simulink model "FieldOrientedControl_Model"  (R2024b)
settings: Solver=FixedStepAuto  StartTime=0.0  StopTime=10.0  FixedStep=1e-07  RelTol=1e-3
InitFcn:
  | clear all;
  | clc;
  | Start_Run;
values from neighbouring files (symbols this model uses):
  dq_decouping_ena = Simulink.Parameter    [FOC_Data.m]
  dq_voltage_ratio = Simulink.Parameter    [FOC_Data.m]
  duty_sat_lower = Simulink.Parameter    [FOC_Data.m]
  duty_sat_upper = Simulink.Parameter    [FOC_Data.m]
  I_s_max = Simulink.Parameter    [FOC_Data.m]
  KI_c = Simulink.Parameter    [FOC_Data.m]
  KI_w = Simulink.Parameter    [FOC_Data.m]
  Kp_c = Simulink.Parameter    [FOC_Data.m]
  Kp_w = Simulink.Parameter    [FOC_Data.m]
  L_d = Simulink.Parameter    [FOC_Data.m]
  L_q = Simulink.Parameter    [FOC_Data.m]
  p = Simulink.Parameter    [FOC_Data.m]
  Psi_p = Simulink.Parameter    [FOC_Data.m]
  rad_s_to_rpm = Simulink.Parameter    [FOC_Data.m]
  sample_time_MIL = Simulink.Parameter    [FOC_Data.m]
  svpwm_ena = Simulink.Parameter    [FOC_Data.m]
  T_limit_Nm = Simulink.Parameter    [FOC_Data.m]
  task_time_mtrctrl = Simulink.Parameter    [FOC_Data.m]
  w_cntrl_reset = Simulink.Parameter    [FOC_Data.m]
  w_m_max = Simulink.Parameter    [FOC_Data.m]
undefined symbols (not defined in the file or in its folder): DiscIntNeverNeededParam, pmsm, PWM_frequency, Ts
libraries: nesl_utility x13, fl_lib x8, simulink x7, ee_lib x5, mcbcontrolslib x2, eeGeneralControl x1, spsPWMGenerator2LevelLib x1, SignalEditorBlockLib x1
settings Model: Creator=Mayur Patil  LastModifiedBy=Mayur Patil

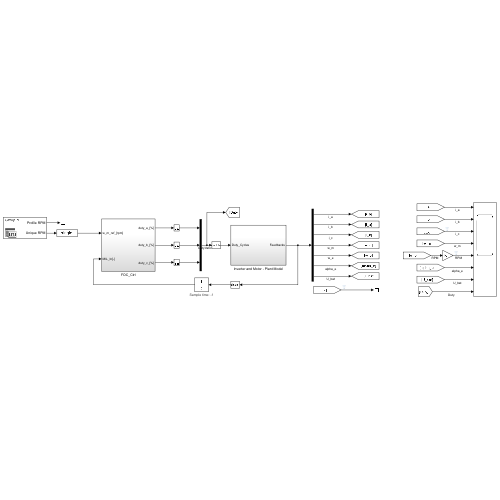
[thumbnail: Simulink's stored preview of the top-level diagram]
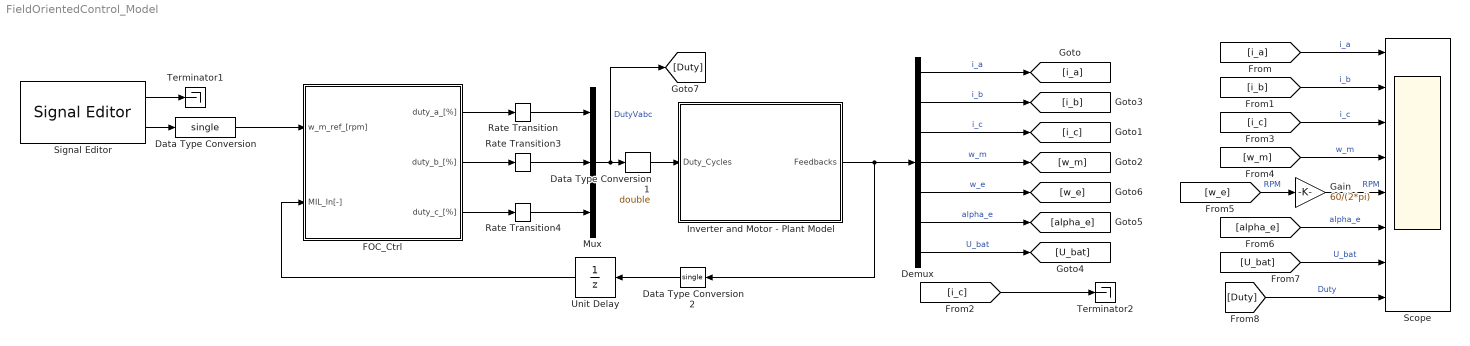
== system FieldOrientedControl_Model ==
  Data Type Conversion : DataTypeConversion  OutDataTypeStr=single  SaturateOnIntegerOverflow=off  RndMeth=Floor
  Data Type Conversion1 : DataTypeConversion  OutDataTypeStr=double  SaturateOnIntegerOverflow=off  RndMeth=Floor
  Data Type Conversion2 : DataTypeConversion  OutDataTypeStr=single  SaturateOnIntegerOverflow=off  RndMeth=Floor
  Demux : Demux  Outputs=7
  FOC_Ctrl : Subsystem
  Gain : Gain  Gain=60/(2*pi)
  Inverter and Motor - Plant Model : Subsystem
  Mux : Mux  Inputs=3
  Rate Transition : RateTransition  OutPortSampleTime=sample_time_MIL
  Rate Transition3 : RateTransition  OutPortSampleTime=sample_time_MIL
  Rate Transition4 : RateTransition  OutPortSampleTime=sample_time_MIL
  Scope : Scope  NumInputPorts=8
  Signal Editor : SignalEditorBlockLib/Signal Editor  FileName=RPM Profile.mat  ActiveScenario=Group_1  ActiveSignal=Profile RPM  IsBus=off  OutputBusObjectStr=Bus: BusObject  SampleTime=0  Interpolate=off  ZeroCross=off  OutputAfterFinalValue=Setting to zero  Unit=inherit  PreserveSignalName=on  ApplySigPropsToAllScenarios=on  ApplySigPropsToAllSignals=off
  Terminator1 : Terminator
  Terminator2 : Terminator
  Unit Delay : UnitDelay  SampleTime=-1  HasFrameUpgradeWarning=on
      settings: AttributesFormatString=Sample time: %<SampleTime>
  wires:
  [i_c] -> Terminator2/1
  [i_b] -> Scope/2  "i_b"
  Mux/1 -> [Duty], Data Type Conversion1/1  "DutyVabc"
  Rate Transition3/1 -> Mux/2
  [i_c] -> Scope/3  "i_c"
  Demux/1 -> [i_a]  "i_a"
  FOC_Ctrl/3(duty_c_[%]) -> Rate Transition4/1
  [w_m] -> Scope/4  "w_m"
  [w_e] -> Gain/1  "RPM"
  [alpha_e] -> Scope/6  "alpha_e"
  Demux/6 -> [alpha_e]  "alpha_e"
  Demux/4 -> [w_m]  "w_m"
  Rate Transition/1 -> Mux/1
  Data Type Conversion/1 -> FOC_Ctrl/1(w_m_ref_[rpm])
  [i_a] -> Scope/1  "i_a"
  Unit Delay/1 -> FOC_Ctrl/2(MIL_In[-])
  Demux/7 -> [U_bat]  "U_bat"
  Demux/2 -> [i_b]  "i_b"
  Signal Editor/1 -> Terminator1/1
  [U_bat] -> Scope/7  "U_bat"
  FOC_Ctrl/2(duty_b_[%]) -> Rate Transition3/1
  Inverter and Motor - Plant Model/1(Feedbacks) -> Data Type Conversion2/1, Demux/1
  Demux/3 -> [i_c]  "i_c"
  Rate Transition4/1 -> Mux/3
  FOC_Ctrl/1(duty_a_[%]) -> Rate Transition/1
  Demux/5 -> [w_e]  "w_e"
  Signal Editor/2 -> Data Type Conversion/1
  Data Type Conversion1/1 -> Inverter and Motor - Plant Model/1(Duty_Cycles)
  Data Type Conversion2/1 -> Unit Delay/1
  [Duty] -> Scope/8  "Duty"
  Gain/1 -> Scope/5  "RPM"

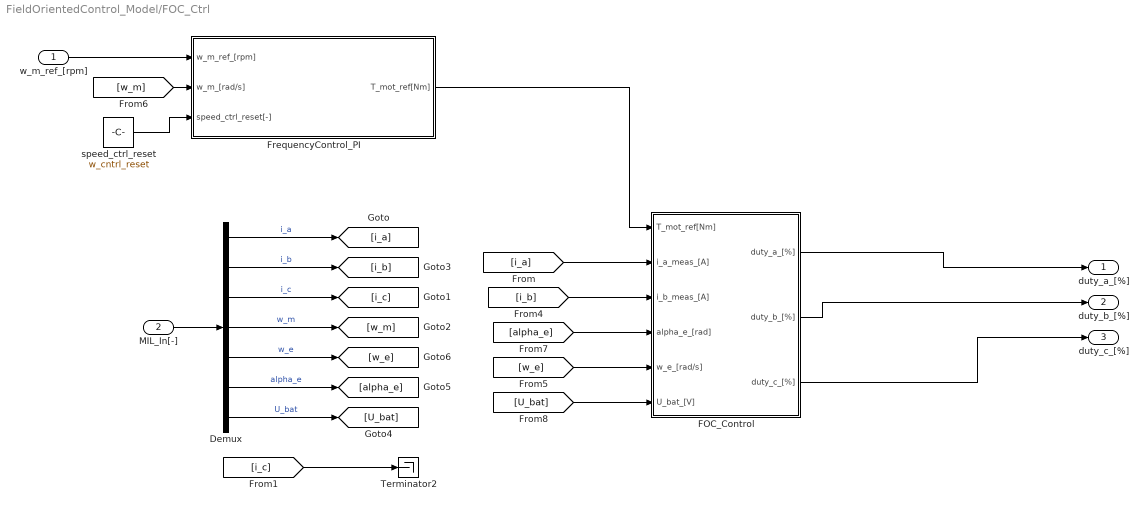
== system FieldOrientedControl_Model/FOC_Ctrl ==
  w_m_ref_[rpm] : Inport
  MIL_In[-] : Inport  Port=2
  Demux : Demux  Outputs=7
  FOC_Control : Subsystem
  FrequencyControl_PI : Subsystem
  Terminator2 : Terminator
  speed_ctrl_reset : Constant  Value=w_cntrl_reset  OutDataTypeStr=boolean
  duty_a_[%] : Outport
  duty_b_[%] : Outport  Port=2
  duty_c_[%] : Outport  Port=3
  wires:
  Demux/2 -> [i_b]  "i_b"
  [alpha_e] -> FOC_Control/4(alpha_e_[rad])
  speed_ctrl_reset/1 -> FrequencyControl_PI/3(speed_ctrl_reset[-])
  FrequencyControl_PI/1(T_mot_ref[Nm]) -> FOC_Control/1(T_mot_ref[Nm])
  Demux/4 -> [w_m]  "w_m"
  [w_m] -> FrequencyControl_PI/2(w_m_[rad/s])
  Demux/6 -> [alpha_e]  "alpha_e"
  w_m_ref_[rpm]/1 -> FrequencyControl_PI/1(w_m_ref_[rpm])
  Demux/1 -> [i_a]  "i_a"
  Demux/7 -> [U_bat]  "U_bat"
  FOC_Control/3(duty_c_[%]) -> duty_c_[%]/1
  [U_bat] -> FOC_Control/6(U_bat_[V])
  Demux/3 -> [i_c]  "i_c"
  [i_a] -> FOC_Control/2(i_a_meas_[A])
  Demux/5 -> [w_e]  "w_e"
  [i_c] -> Terminator2/1
  [i_b] -> FOC_Control/3(i_b_meas_[A])
  [w_e] -> FOC_Control/5(w_e_[rad/s])
  MIL_In[-]/1 -> Demux/1
  FOC_Control/2(duty_b_[%]) -> duty_b_[%]/1
  FOC_Control/1(duty_a_[%]) -> duty_a_[%]/1

== system FieldOrientedControl_Model/Inverter and Motor - Plant Model ==
  Duty_Cycles : Inport
  Inverter : Subsystem  VariantControl=(get_param([bdroot '/InverterSelection'], 'Value') == '1')
  Load_Profile (Torque) : Subsystem
  Feedbacks : Outport  VectorParamsAs1DForOutWhenUnconnected=off
  wires:
  Load_Profile (Torque)/1(Load_Trq) -> Inverter/2(Load)
  Duty_Cycles/1 -> Inverter/1(Vabc_In_PU)
  Inverter/1(Feedback) -> Feedbacks/1

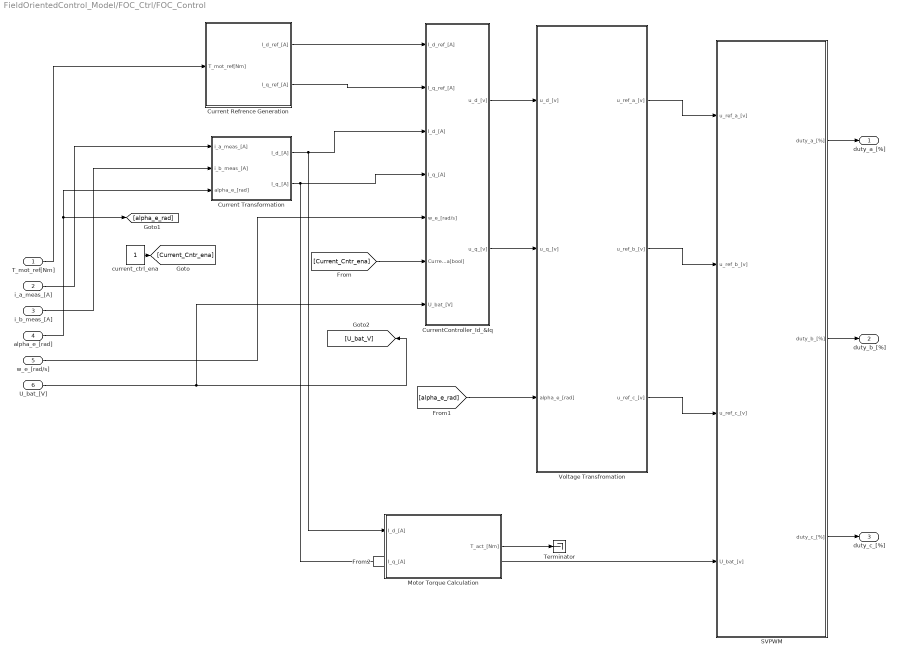
== system FieldOrientedControl_Model/FOC_Ctrl/FOC_Control ==
  T_mot_ref[Nm] : Inport  OutDataTypeStr=single  SampleTime=task_time_mtrctrl
  i_a_meas_[A] : Inport  Port=2  OutDataTypeStr=single  SampleTime=task_time_mtrctrl
  i_b_meas_[A] : Inport  Port=3  OutDataTypeStr=single  SampleTime=task_time_mtrctrl
  alpha_e_[rad] : Inport  Port=4  OutDataTypeStr=single  SampleTime=task_time_mtrctrl
  w_e_[rad/s] : Inport  Port=5  OutDataTypeStr=single  SampleTime=task_time_mtrctrl
  U_bat_[V] : Inport  Port=6  OutDataTypeStr=single  SampleTime=task_time_mtrctrl
  Current Refrence Generation : Subsystem
  Current Transformation : Subsystem
  CurrentController_Id_&Iq : Subsystem
  Motor Torque Calculation : Subsystem
  SVPWM : Subsystem
  Terminator : Terminator
  Voltage Transfromation : Subsystem
  current_ctrl_ena : Constant  OutDataTypeStr=boolean  SampleTime=task_time_mtrctrl
  duty_a_[%] : Outport  OutDataTypeStr=single
  duty_b_[%] : Outport  Port=2  OutDataTypeStr=single
  duty_c_[%] : Outport  Port=3  OutDataTypeStr=single
  wires:
  U_bat_[V]/1 -> [U_bat_V], CurrentController_Id_&Iq/7(U_bat_[V])
  i_b_meas_[A]/1 -> Current Transformation/2(i_b_meas_[A])
  i_a_meas_[A]/1 -> Current Transformation/1(i_a_meas_[A])
  T_mot_ref[Nm]/1 -> Current Refrence Generation/1(T_mot_ref[Nm])
  alpha_e_[rad]/1 -> [alpha_e_rad], Current Transformation/3(alpha_e_[rad])
  CurrentController_Id_&Iq/2(u_q_[v]) -> Voltage Transfromation/2(u_q_[v])
  CurrentController_Id_&Iq/1(u_d_[v]) -> Voltage Transfromation/1(u_d_[v])
  [U_bat_V] -> SVPWM/4(U_bat_[v])
  Current Refrence Generation/1(I_d_ref_[A]) -> CurrentController_Id_&Iq/1(I_d_ref_[A])
  w_e_[rad/s]/1 -> CurrentController_Id_&Iq/5(w_e_[rad/s])
  Current Transformation/2(I_q_[A]) -> CurrentController_Id_&Iq/4(I_q_[A]), Motor Torque Calculation/2(I_q_[A])
  Motor Torque Calculation/1(T_act_[Nm]) -> Terminator/1
  Current Refrence Generation/2(I_q_ref_[A]) -> CurrentController_Id_&Iq/2(I_q_ref_[A])
  [alpha_e_rad] -> Voltage Transfromation/3(alpha_e_[rad])
  Current Transformation/1(I_d_[A]) -> CurrentController_Id_&Iq/3(I_d_[A]), Motor Torque Calculation/1(I_d_[A])
  current_ctrl_ena/1 -> [Current_Cntr_ena]
  [Current_Cntr_ena] -> CurrentController_Id_&Iq/6(Current_Cntr_ena[bool])
  SVPWM/1(duty_a_[%]) -> duty_a_[%]/1
  SVPWM/2(duty_b_[%]) -> duty_b_[%]/1
  SVPWM/3(duty_c_[%]) -> duty_c_[%]/1
  Voltage Transfromation/1(u_ref_a_[v]) -> SVPWM/1(u_ref_a_[v])
  Voltage Transfromation/2(u_ref_b_[v]) -> SVPWM/2(u_ref_b_[v])
  Voltage Transfromation/3(u_ref_c_[v]) -> SVPWM/3(u_ref_c_[v])

== system FieldOrientedControl_Model/FOC_Ctrl/FrequencyControl_PI ==
  w_m_ref_[rpm] : Inport
  w_m_[rad/s] : Inport  Port=2
  speed_ctrl_reset[-] : Inport  Port=3
  KI_rpm : Constant  Value=KI_w  OutDataTypeStr=single
  KP_rpm : Constant  Value=Kp_w  OutDataTypeStr=single
  PI regulator : Subsystem
  Saturation Dynamic : simulink/Discontinuities/Saturation Dynamic  OutMin=[]  OutMax=[]  OutDataTypeStr=Inherit: Same as second input  OutDataType=fixdt(1, 16)  OutScaling=2^-10  RndMeth=Simplest  DoSatur=off
  Subtract : Sum  Inputs=+-  RndMeth=Simplest  SaturateOnIntegerOverflow=on
  T_e_limit_Nm : Constant  Value=T_limit_Nm
  Unary Minus : UnaryMinus  SaturateOnIntegerOverflow=on
  rad/s_to_rpm : Gain  Gain=rad_s_to_rpm  RndMeth=Simplest  SaturateOnIntegerOverflow=on
  w_m_max : Constant  Value=w_m_max
  T_mot_ref[Nm] : Outport
  wires:
  KI_rpm/1 -> PI regulator/3(I)
  KP_rpm/1 -> PI regulator/2(P)
  w_m_max/1 -> Saturation Dynamic/1, Unary Minus/1
  T_e_limit_Nm/1 -> PI regulator/4(OutputLimit)
  w_m_ref_[rpm]/1 -> Saturation Dynamic/2
  PI regulator/1(PI_Daw_Out) -> T_mot_ref[Nm]/1  "T_mot_ref_sat"
  speed_ctrl_reset[-]/1 -> PI regulator/5(ResetExt)
  Saturation Dynamic/1 -> Subtract/1  "w_m_ref_sat_rpm"
  Subtract/1 -> PI regulator/1(Error)  "w_m_err_rpm"
  Unary Minus/1 -> Saturation Dynamic/3
  w_m_[rad/s]/1 -> rad/s_to_rpm/1
  rad/s_to_rpm/1 -> Subtract/2  "w_m_rpm"

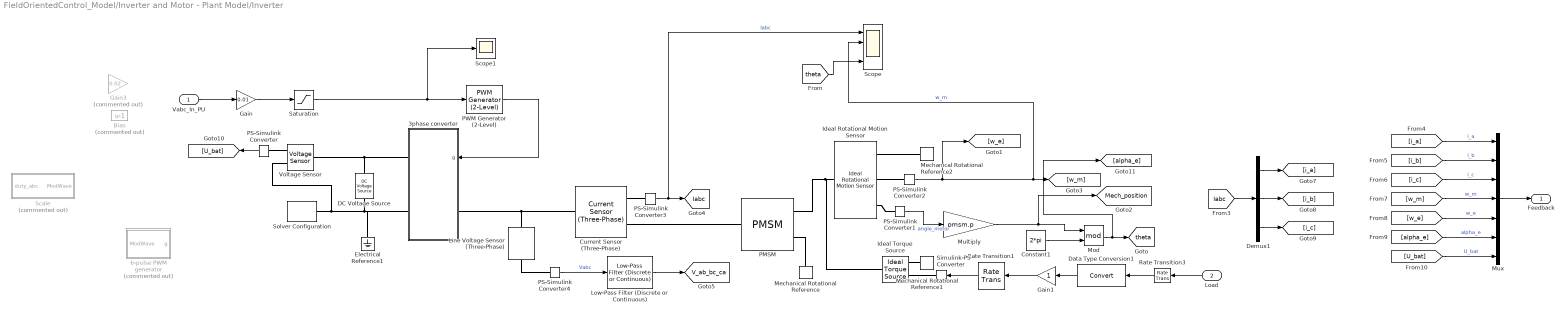
== system FieldOrientedControl_Model/Inverter and Motor - Plant Model/Inverter ==
  Vabc_In_PU : Inport
  Load : Inport  Port=2
  3phase converter : Subsystem
  6-pulse PWM generator : Subsystem  Commented=on  mask{fs=PWM_frequency}
      mask prompts: fs "Carrier Frequency (Hz)"
  Bias : Bias  Commented=on  Bias=-1  SaturateOnIntegerOverflow=off
  Constant1 : Constant  Value=2*pi
  Current Sensor (Three-Phase) : ee_lib/Sensors & Transducers/Current Sensor (Three-Phase)
  DC Voltage Source : fl_lib/Electrical/Electrical Sources/DC Voltage Source  v0=inverter.V_dc V
  Data Type Conversion1 : DataTypeConversion  SaturateOnIntegerOverflow=off  RndMeth=Floor
  Demux1 : Demux  Outputs=3
  Electrical Reference1 : fl_lib/Electrical/Electrical Elements/Electrical Reference
  Gain : Gain  Gain=0.01
  Gain1 : Gain
  Gain3 : Gain  Commented=on  Gain=0.02
  Ideal Rotational Motion Sensor : fl_lib/Mechanical/Mechanical Sensors/Ideal Rotational Motion Sensor  reference=foundation.enum.MeasurementReference.difference  acceleration_port=false  velocity_port=true  position_port=true  wrap_angle=simscape.enum.onoff.off  offset=0 rad
  Ideal Torque Source : fl_lib/Mechanical/Mechanical Sources/Ideal Torque Source
  Line Voltage Sensor (Three-Phase) : ee_lib/Sensors & Transducers/Line Voltage Sensor (Three-Phase)
  Low-Pass Filter (Discrete or Continuous) : eeGeneralControl/Low-Pass Filter (Discrete or Continuous)  K=1  T=5e-4  B=inf  A=-inf  init_option=Inherited from block input  x0=0  Ts=-1
  Mechanical Rotational Reference : fl_lib/Mechanical/Rotational Elements/Mechanical Rotational Reference
  Mechanical Rotational Reference1 : fl_lib/Mechanical/Rotational Elements/Mechanical Rotational Reference
  Mechanical Rotational Reference2 : fl_lib/Mechanical/Rotational Elements/Mechanical Rotational Reference
  Mod : Math  Operator=mod
  Multiply : Gain  Gain=pmsm.p
  Mux : Mux  Inputs=7
  PMSM : ee_lib/Electromechanical/Permanent Magnet/PMSM  port_option=ee.enum.threePhasePort.composite  winding_type=ee.enum.statorconnection.wye  machine_param=ee.enum.pmsm.parameterization.constant  nPolePairs=pmsm.p  pmflux_param=ee.enum.pmflux.fluxlinkage  pm_flux_linkage=pmsm.FluxPM Wb  torque_constant=0.18 N*m/A  back_emf_constant=0.18 V/(rad/s)  stator_param=ee.enum.statorparam.LdLqL0  Ld=pmsm.Ld H  Lq=pmsm.Lq H  idVec=[-200, 0, 200] A  iqVec=[-200, 0, 200] A  LdMatrix=0.0002 * ones(3, 3) H  LqMatrix=0.0002 * ones(3, 3) H  PmMatrix=0.1 * ones(3, 3) Wb  ktMatrix=0.18 * ones(3, 3) N*m/A  keMatrix=0.18 * ones(3, 3) V/(rad/s)  L0=0 H  Ls=0.0002 H  Lm=-0.00002 H  Ms=0.00002 H  Rs=pmsm.Rs Ohm  zero_sequence=ee.enum.park.zerosequence.exclude  axes_param=ee.enum.rotorangle.daxis  loss_param=ee.enum.ironloss.none  losses_oc=[0, 0, 0] W  losses_sc=[0, 0, 0] W  f_losses=60 Hz  Isc_losses=95 A  J=pmsm.J kg*m^2  lam=pmsm.B N*m/(rad/s)  i_d_specify=off  i_d_priority=None  i_d=0 A  i_d_nominal_specify=off  i_d_nominal_value=1  i_d_nominal_unit=A  i_q_specify=off  i_q_priority=None  i_q=0 A  i_q_nominal_specify=off  i_q_nominal_value=1  i_q_nominal_unit=A  torque_specify=off  torque_priority=None  torque=0 N*m  torque_nominal_specify=off  torque_nominal_value=1  torque_nominal_unit=N*m  angular_velocity_specify=off  angular_velocity_priority=High  angular_velocity=0 rpm  angular_velocity_nominal_specify=off  angular_velocity_nominal_value=1  angular_velocity_nominal_unit=rpm  angular_position_specify=off  angular_position_priority=High  angular_position=0 deg  angular_position_nominal_specify=off  angular_position_nominal_value=1  angular_position_nominal_unit=deg  alpha=3.93e-3 1/K  alpha_flux=-0.001 1/K  Tmeas=298.15 K  stator_thermal_mass=100 J/K  rotor_thermal_mass=200 J/K  Rm_percent_rotor=90  Rd_percent_rotor=30  temperatureA_specify=off  temperatureA_priority=High  temperatureA=25 degC  temperatureA_nominal_specify=off  temperatureA_nominal_value=1  temperatureA_nominal_unit=degC  temperatureB_specify=off  temperatureB_priority=High  temperatureB=25 degC  temperatureB_nominal_specify=off  temperatureB_nominal_value=1  temperatureB_nominal_unit=degC  temperatureC_specify=off  temperatureC_priority=High  temperatureC=25 degC  temperatureC_nominal_specify=off  temperatureC_nominal_value=1  temperatureC_nominal_unit=degC  temperatureR_specify=off  temperatureR_priority=High  temperatureR=25 degC  temperatureR_nominal_specify=off  temperatureR_nominal_value=1  temperatureR_nominal_unit=degC
      settings: InternalSimscapePortConfiguration="{\"Bottom\":[],\"Left\":[{\"id\":\"N\",\"label\":\"~\",\"type\":\"foundation.electrical.three_phase\"}],\"Right\":[{\"id\":\"R\",\"label\":\"R\",\"type\":\"foundation.mechanical.rotational.rotational\"},{\"id\":\"C\",\"label\":\"C\",\"type\":\"foundation.mechanical.rotational.rotational\"}],\"Top\":[]}"
  PS-Simulink Converter : nesl_utility/PS-Simulink Converter  PhysicalDomain=network_engine_domain  SubClassName=ps_output  LeftPortType=input  RightPortType=output  PseudoPeriodic=off  Frequencies=[]  VectorFormat=inherit  Unit=inherit  AffineConversion=off
  PS-Simulink Converter1 : nesl_utility/PS-Simulink Converter  PhysicalDomain=network_engine_domain  SubClassName=ps_output  LeftPortType=input  RightPortType=output  PseudoPeriodic=off  Frequencies=[]  VectorFormat=1-D array  Unit=rad  AffineConversion=off
  PS-Simulink Converter2 : nesl_utility/PS-Simulink Converter  PhysicalDomain=network_engine_domain  SubClassName=ps_output  LeftPortType=input  RightPortType=output  PseudoPeriodic=off  Frequencies=[]  VectorFormat=1-D array  Unit=rad/s  AffineConversion=off
  PS-Simulink Converter3 : nesl_utility/PS-Simulink Converter  PhysicalDomain=network_engine_domain  SubClassName=ps_output  LeftPortType=input  RightPortType=output  PseudoPeriodic=off  Frequencies=[]  VectorFormat=1-D array  Unit=inherit  AffineConversion=off
  PS-Simulink Converter4 : nesl_utility/PS-Simulink Converter  PhysicalDomain=network_engine_domain  SubClassName=ps_output  LeftPortType=input  RightPortType=output  PseudoPeriodic=off  Frequencies=[]  VectorFormat=1-D array  Unit=inherit  AffineConversion=off
  PWM Generator (2-Level) : spsPWMGenerator2LevelLib/PWM Generator (2-Level)  ModulatorType=Three-phase bridge (6 pulses)  ModulatorMode=Unsynchronized  Fc=12000  Pc=90  nF=27  MinMax="[ 0  1 ]"  SamplingTechnique=Natural  ModulatingSignals=off  m=0.8  Freq=60  Phase=0  Ts=sample_time_MIL  ShowCarrierOutport=off
  Rate Transition1 : RateTransition  OutPortSampleTime=Ts
  Rate Transition3 : RateTransition  Deterministic=off  OutPortSampleTime=Ts
  Saturation : Saturate  UpperLimit=1  LowerLimit=0
  Scale : Subsystem  Commented=on
  Scope : Scope  NumInputPorts=4
  Scope1 : Scope
  Simulink-PS Converter : nesl_utility/Simulink-PS Converter  PhysicalDomain=network_engine_domain  SubClassName=ps_input  LeftPortType=input  RightPortType=output  PseudoPeriodic=off  Frequencies=[]  NoiseDistribution=none  NoiseParameters=[]  Unit=N*m  AffineConversion=off  FilteringAndDerivatives=provide  SimscapeFilterOrder=1  InputFilterTimeConstant=0.001  UdotUserProvided=0
  Solver Configuration : nesl_utility/Solver Configuration  PhysicalDomain=network_engine_domain  SubClassName=solver  LeftPortType=input  RightPortType=generic  Tones=[]  Harmonics=[]  SimulateNoise=off  Profile=off  UseLocalSampling=off  EnableSwitchedLinearOptims=on  FrequencyDomain=off  UseCCode=off  RelTol=0.001  AbsTol=1e-06  MinStep=1e-09  ToWorkspace=off  RevertToSquareIcSolve=off  NumHomotopyIterations=100  PhasorMode=off  PhasorModeNumHarmonics=1  ConsistencySolver=NEWTON_FTOL  IndexReductionMethod=DerivativeReplacement  DoDC=off  ResidualTolerance=1e-09  ConsistencyTolSource=GLOBAL  ConsistencyAbsTol=0.001  ConsistencyRelTol=0.001  ConsistencyTolFactor=0.001  UseLocalSolver=on  LocalSolverChoice=NE_BACKWARD_EULER_ADVANCER  ResolveIndetEquations=on  FunctionEvalNumThread=1  LocalSolverSampleTime=1e-7  DoFixedCost=off  MaxNonlinIter=1  MaxModeIter=2  ComputeImpulses=off  ImpulseIterations=1  LinearAlgebra=Sparse  LinearAlgebraNumThread=0  EquationFormulation=NE_TIME_EF  DelaysMemoryBudget=1024  AutomaticFiltering=off  FilteringTimeConstant=0.001  PartitionStorageMethod=AS_NEEDED  PartitionMemoryBudget=1024  PartitionMethod=ROBUST  MultibodyUseLocalSolver=off  MultibodyLocalSolverChoice=ODE1  MultibodyLocalSolverSampleTime=0.001
  Voltage Sensor : fl_lib/Electrical/Electrical Sensors/Voltage Sensor
  Feedback : Outport
  tag scope: Iabc=global, Mech_position=global, V_ab_bc_ca=global, theta=global
  wires:
  Load/1 -> Rate Transition3/1
  Vabc_In_PU/1 -> Gain/1
  PWM Generator (2-Level)/1 -> 3phase converter/1(g)
  Demux1/1 -> [i_a]
  Demux1/2 -> [i_b]
  Demux1/3 -> [i_c]
  [Iabc] -> Demux1/1
  PS-Simulink Converter/1 -> [U_bat]
  [i_a] -> Mux/1  "i_a"
  [i_b] -> Mux/2  "i_b"
  [i_c] -> Mux/3  "i_c"
  [w_m] -> Mux/4  "w_m"
  [w_e] -> Mux/5  "w_e"
  [alpha_e] -> Mux/6  "alpha_e"
  [U_bat] -> Mux/7  "U_bat"
  Mux/1 -> Feedback/1
  Multiply/1 -> [Mech_position], Mod/1
  Mod/1 -> [alpha_e], [theta]
  Constant1/1 -> Mod/2
  PS-Simulink Converter1/1 -> Multiply/1  "angle_motor"
  PS-Simulink Converter2/1 -> Scope/2, [w_m], [w_e]  "w_m"
  Rate Transition3/1 -> Data Type Conversion1/1
  Data Type Conversion1/1 -> Gain1/1
  Rate Transition1/1 -> Simulink-PS Converter/1
  Gain1/1 -> Rate Transition1/1
  Low-Pass Filter (Discrete or Continuous)/1 -> [V_ab_bc_ca]
  PS-Simulink Converter3/1 -> Scope/1, [Iabc]  "Iabc"
  PS-Simulink Converter4/1 -> Low-Pass Filter (Discrete or Continuous)/1  "Vabc"
  [theta] -> Scope/4
  Gain/1 -> Saturation/1
  Saturation/1 -> Scope1/1, PWM Generator (2-Level)/1
  connections:
  Solver Configuration/RConn1 -- Electrical Reference1/LConn1 -- 3phase converter/RConn2 -- DC Voltage Source/RConn1 -- Voltage Sensor/RConn2
  Current Sensor (Three-Phase)/RConn2 -- PMSM/LConn1
  Line Voltage Sensor (Three-Phase)/LConn1 -- 3phase converter/LConn1 -- Current Sensor (Three-Phase)/LConn1
  Mechanical Rotational Reference/LConn1 -- PMSM/RConn2
  Ideal Torque Source/LConn1 -- PMSM/RConn1 -- Ideal Rotational Motion Sensor/LConn1
  DC Voltage Source/LConn1 -- Voltage Sensor/LConn1 -- 3phase converter/RConn1
  Voltage Sensor/RConn1 -- PS-Simulink Converter/LConn1
  Mechanical Rotational Reference2/LConn1 -- Ideal Rotational Motion Sensor/RConn1
  PS-Simulink Converter1/LConn1 -- Ideal Rotational Motion Sensor/RConn3
  Ideal Rotational Motion Sensor/RConn2 -- PS-Simulink Converter2/LConn1
  Simulink-PS Converter/RConn1 -- Ideal Torque Source/RConn1
  Mechanical Rotational Reference1/LConn1 -- Ideal Torque Source/RConn2
  PS-Simulink Converter4/LConn1 -- Line Voltage Sensor (Three-Phase)/RConn1
  Current Sensor (Three-Phase)/RConn1 -- PS-Simulink Converter3/LConn1

== system FieldOrientedControl_Model/Inverter and Motor - Plant Model/Load_Profile (Torque) ==
  Data Type Conversion : DataTypeConversion  OutDataTypeStr=single  SaturateOnIntegerOverflow=off  RndMeth=Floor
  IIR Filter : mcbcontrolslib/IIR Filter  VariantControl=Low Pass Filter  VariantSelect=Low-pass  FilterConstantInputType=Specify via dialog  Filter_constant=0.01  advancedSettings=off  Ts=50e-6  cutOff_freq=32.1525
  T_load : Constant  Value=0  OutDataTypeStr=double  SampleTime=Ts
  Load_Trq : Outport  VectorParamsAs1DForOutWhenUnconnected=off
  wires:
  T_load/1 -> Data Type Conversion/1
  Data Type Conversion/1 -> IIR Filter/1
  IIR Filter/1 -> Load_Trq/1

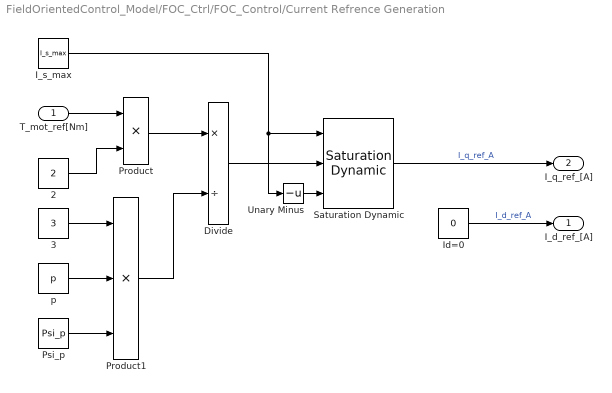
== system FieldOrientedControl_Model/FOC_Ctrl/FOC_Control/Current Refrence Generation ==
  T_mot_ref[Nm] : Inport
  2 : Constant  Value=2
  3 : Constant  Value=3
  Divide : Product  Inputs=*/
  I_s_max : Constant  Value=I_s_max
  Id=0 : Constant  Value=0
  Product : Product
  Product1 : Product  Inputs=3
  Psi_p : Constant  Value=Psi_p
  Saturation Dynamic : simulink/Discontinuities/Saturation Dynamic  OutMin=[]  OutMax=[]  OutDataTypeStr=Inherit: Same as second input  OutDataType=fixdt(1, 16)  OutScaling=2^-10  DoSatur=off
  Unary Minus : UnaryMinus
  p : Constant  Value=p
  I_d_ref_[A] : Outport
  I_q_ref_[A] : Outport  Port=2
  wires:
  T_mot_ref[Nm]/1 -> Product/1
  2/1 -> Product/2
  3/1 -> Product1/1
  p/1 -> Product1/2
  Psi_p/1 -> Product1/3
  Product/1 -> Divide/1
  Product1/1 -> Divide/2
  Divide/1 -> Saturation Dynamic/2
  Saturation Dynamic/1 -> I_q_ref_[A]/1  "I_q_ref_A"
  I_s_max/1 -> Saturation Dynamic/1, Unary Minus/1
  Unary Minus/1 -> Saturation Dynamic/3
  Id=0/1 -> I_d_ref_[A]/1  "I_d_ref_A"

== system FieldOrientedControl_Model/FOC_Ctrl/FOC_Control/Current Transformation ==
  i_a_meas_[A] : Inport
  i_b_meas_[A] : Inport  Port=2
  alpha_e_[rad] : Inport  Port=3
  Clark Transformation : Subsystem
  Park Transformation : Subsystem
  I_d_[A] : Outport
  I_q_[A] : Outport  Port=2
  wires:
  i_a_meas_[A]/1 -> Clark Transformation/1(i_a_meas_[A])
  i_b_meas_[A]/1 -> Clark Transformation/2(i_b_meas_[A])
  Clark Transformation/1(i_x_[A]) -> Park Transformation/1(i_x_[A])  "i_x_mean_A"
  Clark Transformation/2(i_y_[A]) -> Park Transformation/2(i_y_[A])  "i_y_mean_A"
  alpha_e_[rad]/1 -> Park Transformation/3(alpha_e_[rad])
  Park Transformation/1(I_d_[A]) -> I_d_[A]/1  "id_mean_A"
  Park Transformation/2(I_q_[A]) -> I_q_[A]/1  "iq_mean_A"

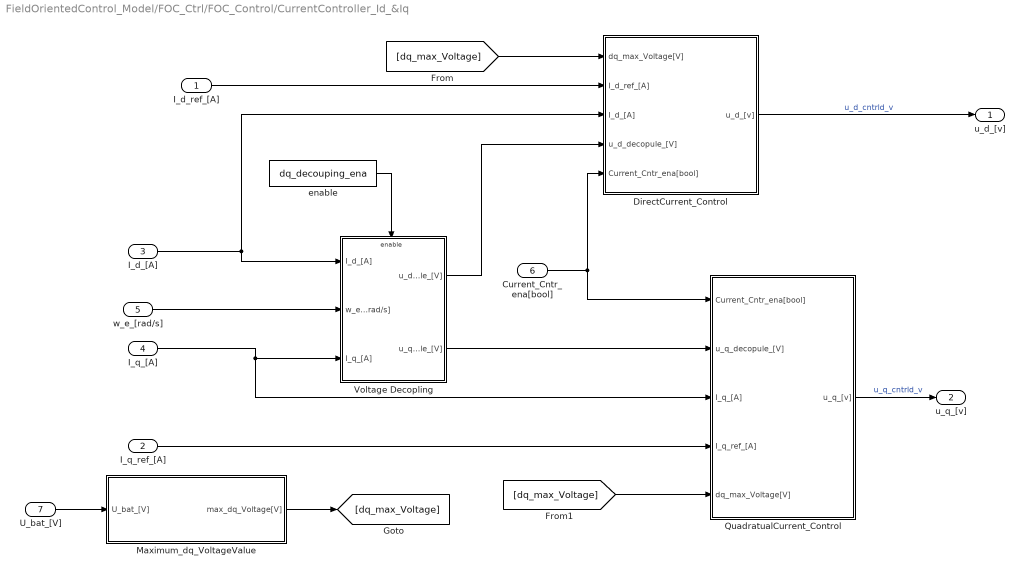
== system FieldOrientedControl_Model/FOC_Ctrl/FOC_Control/CurrentController_Id_&Iq ==
  I_d_ref_[A] : Inport
  I_q_ref_[A] : Inport  Port=2
  I_d_[A] : Inport  Port=3
  I_q_[A] : Inport  Port=4
  w_e_[rad/s] : Inport  Port=5
  Current_Cntr_ena[bool] : Inport  Port=6
  U_bat_[V] : Inport  Port=7
  DirectCurrent_Control : Subsystem
  Maximum_dq_VoltageValue : Subsystem
  QuadratualCurrent_Control : Subsystem
  Voltage Decopling : Subsystem
  enable : Constant  Value=dq_decouping_ena
  u_d_[v] : Outport
  u_q_[v] : Outport  Port=2
  wires:
  I_q_[A]/1 -> QuadratualCurrent_Control/3(I_q_[A]), Voltage Decopling/3(I_q_[A])
  I_d_[A]/1 -> DirectCurrent_Control/3(I_d_[A]), Voltage Decopling/1(I_d_[A])
  w_e_[rad/s]/1 -> Voltage Decopling/2(w_e_[rad/s])
  I_d_ref_[A]/1 -> DirectCurrent_Control/2(I_d_ref_[A])
  Current_Cntr_ena[bool]/1 -> QuadratualCurrent_Control/1(Current_Cntr_ena[bool]), DirectCurrent_Control/5(Current_Cntr_ena[bool])
  Voltage Decopling/1(u_d_decopule_[V]) -> DirectCurrent_Control/4(u_d_decopule_[V])
  U_bat_[V]/1 -> Maximum_dq_VoltageValue/1(U_bat_[V])
  Maximum_dq_VoltageValue/1(max_dq_Voltage[V]) -> [dq_max_Voltage]
  [dq_max_Voltage] -> DirectCurrent_Control/1(dq_max_Voltage[V])
  DirectCurrent_Control/1(u_d_[v]) -> u_d_[v]/1  "u_d_cntrld_v"
  [dq_max_Voltage] -> QuadratualCurrent_Control/5(dq_max_Voltage[V])
  QuadratualCurrent_Control/1(u_q_[v]) -> u_q_[v]/1  "u_q_cntrld_v"
  Voltage Decopling/2(u_q_decopule_[V]) -> QuadratualCurrent_Control/2(u_q_decopule_[V])
  I_q_ref_[A]/1 -> QuadratualCurrent_Control/4(I_q_ref_[A])
  enable/1 -> Voltage Decopling/Enable

== system FieldOrientedControl_Model/FOC_Ctrl/FOC_Control/Motor Torque Calculation ==
  I_d_[A] : Inport
  I_q_[A] : Inport  Port=2
  Add : Sum  Inputs=+-
  Add1 : Sum
  Constant : Constant  Value=L_d
  Constant1 : Constant  Value=L_q
  Constant2 : Constant  Value=p
  Constant3 : Constant  Value=Psi_p
  Constant4 : Constant  Value=3/2
  Product : Product  Inputs=3
  Product1 : Product
  Product2 : Product  Inputs=3
  T_act_[Nm] : Outport
  wires:
  Constant/1 -> Add/1
  Constant1/1 -> Add/2
  Add/1 -> Product/1
  I_d_[A]/1 -> Product/2
  I_q_[A]/1 -> Product1/1, Product/3
  Constant3/1 -> Product1/2
  Product/1 -> Add1/1
  Product1/1 -> Add1/2
  Add1/1 -> Product2/1
  Constant2/1 -> Product2/2
  Constant4/1 -> Product2/3
  Product2/1 -> T_act_[Nm]/1  "T_act_Nm"

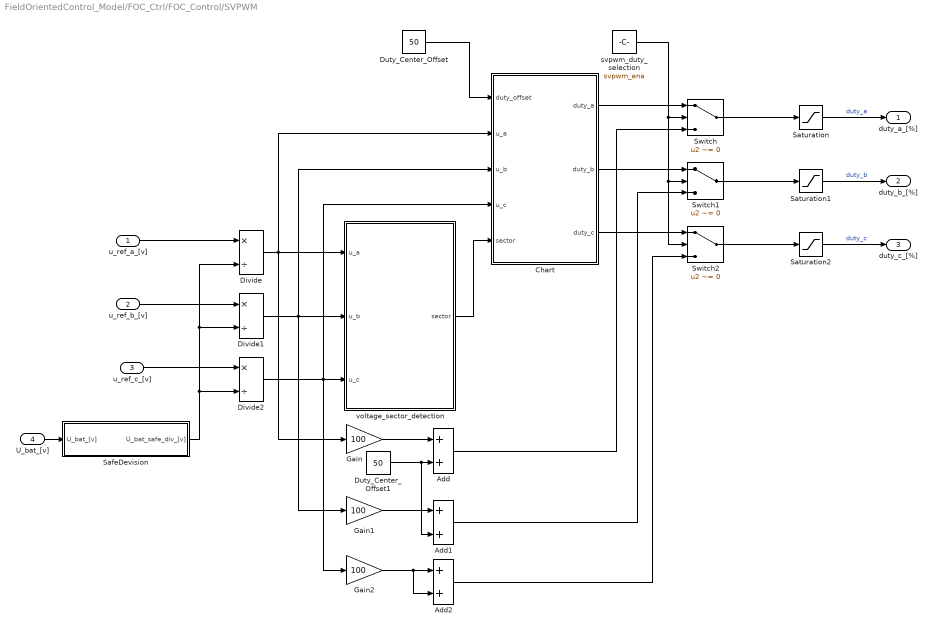
== system FieldOrientedControl_Model/FOC_Ctrl/FOC_Control/SVPWM ==
  u_ref_a_[v] : Inport
  u_ref_b_[v] : Inport  Port=2
  u_ref_c_[v] : Inport  Port=3
  U_bat_[v] : Inport  Port=4
  Add : Sum
  Add1 : Sum
  Add2 : Sum
  Chart : Stateflow chart  TreatAsAtomicUnit=on
  Divide : Product  Inputs=*/
  Divide1 : Product  Inputs=*/
  Divide2 : Product  Inputs=*/
  Duty_Center_Offset : Constant  Value=50
  Duty_Center_Offset1 : Constant  Value=50
  Gain : Gain  Gain=100
  Gain1 : Gain  Gain=100
  Gain2 : Gain  Gain=100
  SafeDevision : Subsystem
  Saturation : Saturate  UpperLimit=duty_sat_upper  LowerLimit=duty_sat_lower
  Saturation1 : Saturate  UpperLimit=duty_sat_upper  LowerLimit=duty_sat_lower
  Saturation2 : Saturate  UpperLimit=duty_sat_upper  LowerLimit=duty_sat_lower
  Switch : Switch  Criteria=u2 ~= 0  SaturateOnIntegerOverflow=off  InputSameDT=off
  Switch1 : Switch  Criteria=u2 ~= 0  SaturateOnIntegerOverflow=off  InputSameDT=off
  Switch2 : Switch  Criteria=u2 ~= 0  SaturateOnIntegerOverflow=off  InputSameDT=off
  svpwm_duty_selection : Constant  Value=svpwm_ena
  voltage_sector_detection : Stateflow chart  TreatAsAtomicUnit=on
  duty_a_[%] : Outport
  duty_b_[%] : Outport  Port=2
  duty_c_[%] : Outport  Port=3
  wires:
  U_bat_[v]/1 -> SafeDevision/1(U_bat_[v])
  u_ref_a_[v]/1 -> Divide/1
  u_ref_b_[v]/1 -> Divide1/1
  u_ref_c_[v]/1 -> Divide2/1
  SafeDevision/1(U_bat_safe_div_[v]) -> Divide2/2, Divide1/2, Divide/2
  Divide/1 -> Gain/1, voltage_sector_detection/1(u_a), Chart/2(u_a)
  Divide1/1 -> Gain1/1, voltage_sector_detection/2(u_b), Chart/3(u_b)
  Divide2/1 -> Gain2/1, Chart/4(u_c), voltage_sector_detection/3(u_c)
  voltage_sector_detection/1(sector) -> Chart/5(sector)
  Duty_Center_Offset/1 -> Chart/1(duty_offset)
  Gain/1 -> Add/1
  Duty_Center_Offset1/1 -> Add1/2, Add/2
  Gain1/1 -> Add1/1
  Gain2/1 -> Add2/2, Add2/1
  Chart/1(duty_a) -> Switch/1
  Chart/2(duty_b) -> Switch1/1
  Chart/3(duty_c) -> Switch2/1
  Add/1 -> Switch/3
  Add1/1 -> Switch1/3
  Add2/1 -> Switch2/3
  svpwm_duty_selection/1 -> Switch2/2, Switch1/2, Switch/2
  Switch/1 -> Saturation/1
  Saturation/1 -> duty_a_[%]/1  "duty_a"
  Switch1/1 -> Saturation1/1
  Saturation1/1 -> duty_b_[%]/1  "duty_b"
  Switch2/1 -> Saturation2/1
  Saturation2/1 -> duty_c_[%]/1  "duty_c"

== system FieldOrientedControl_Model/FOC_Ctrl/FOC_Control/Voltage Transfromation ==
  u_d_[v] : Inport
  u_q_[v] : Inport  Port=2
  alpha_e_[rad] : Inport  Port=3
  Data Type Conversion : DataTypeConversion  OutDataTypeStr=single  SaturateOnIntegerOverflow=off  RndMeth=Floor
  Data Type Conversion1 : DataTypeConversion  OutDataTypeStr=single  SaturateOnIntegerOverflow=off  RndMeth=Floor
  "Inverse Clark Transformation " : Subsystem
  Inverse Park Transformation : Subsystem
  PWM Reference Generator : mcbcontrolslib/PWM Reference Generator  inSignal=Valphabeta  modType=SVM: space vector modulation
      settings: LibrarySourceBlock=mcbhdllib/Controls/Math Transforms/PWM Reference Generator
  Scope : Scope  NumInputPorts=3
  u_ref_a_[v] : Outport
  u_ref_b_[v] : Outport  Port=2
  u_ref_c_[v] : Outport  Port=3
  wires:
  u_d_[v]/1 -> Inverse Park Transformation/1(u_d_[v])
  u_q_[v]/1 -> Inverse Park Transformation/2(u_q_[v])
  alpha_e_[rad]/1 -> Inverse Park Transformation/3(alpha_e_[rad])
  Inverse Park Transformation/1(u_x_[v]) -> Data Type Conversion/1, "Inverse Clark Transformation "/1(u_x_[v])  "u_x_v"
  Inverse Park Transformation/2(u_y_[v]) -> Data Type Conversion1/1, "Inverse Clark Transformation "/2(u_y_[v])  "u_y_v"
  "Inverse Clark Transformation "/1(u_ref_a_[v]) -> u_ref_a_[v]/1  "u_ref_a_V"
  "Inverse Clark Transformation "/2(u_ref_b_[v]) -> u_ref_b_[v]/1  "u_ref_b_V"
  "Inverse Clark Transformation "/3(u_ref_c_[v]) -> u_ref_c_[v]/1  "u_ref_c_V"
  Data Type Conversion/1 -> PWM Reference Generator/1
  Data Type Conversion1/1 -> PWM Reference Generator/2
  PWM Reference Generator/1 -> Scope/1
  PWM Reference Generator/2 -> Scope/2
  PWM Reference Generator/3 -> Scope/3

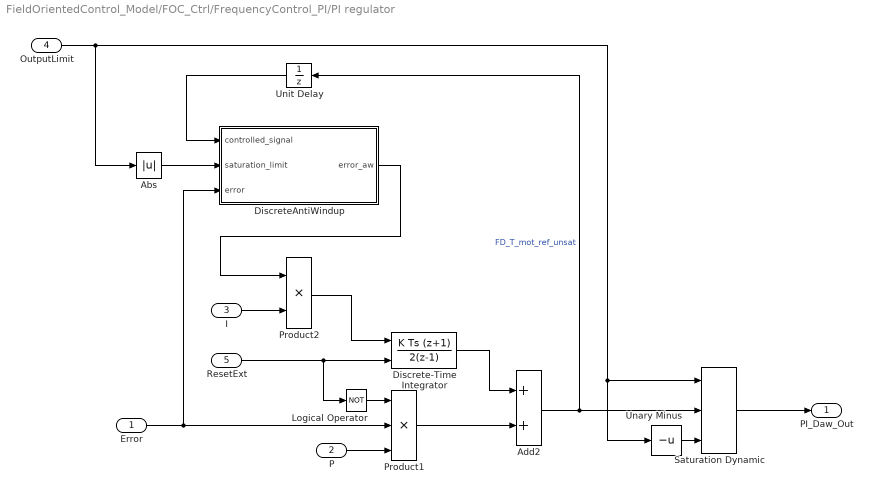
== system FieldOrientedControl_Model/FOC_Ctrl/FrequencyControl_PI/PI regulator ==
  Error : Inport
  P : Inport  Port=2
  I : Inport  Port=3
  OutputLimit : Inport  Port=4
  ResetExt : Inport  Port=5
  Abs : Abs  RndMeth=Simplest
  Add2 : Sum  RndMeth=Simplest  SaturateOnIntegerOverflow=on
  Discrete-Time Integrator : DiscreteIntegrator  IntegratorMethod=Integration: Trapezoidal  ExternalReset=level  SampleTime=-1  RndMeth=Simplest  SaturateOnIntegerOverflow=on  ICPrevOutput=DiscIntNeverNeededParam  ICPrevScaledInput=DiscIntNeverNeededParam
  DiscreteAntiWindup : Subsystem
  Logical Operator : Logic  Operator=NOT  AllPortsSameDT=off  OutDataTypeStr=boolean
  Product1 : Product  Inputs=3  RndMeth=Simplest  SaturateOnIntegerOverflow=on
  Product2 : Product  RndMeth=Simplest  SaturateOnIntegerOverflow=on
  Saturation Dynamic : simulink/Discontinuities/Saturation Dynamic  OutMin=[]  OutMax=[]  OutDataTypeStr=Inherit: Same as second input  OutDataType=fixdt(1, 16)  OutScaling=2^-10  RndMeth=Simplest  DoSatur=off
  Unary Minus : UnaryMinus  SaturateOnIntegerOverflow=on
  Unit Delay : UnitDelay  SampleTime=-1  HasFrameUpgradeWarning=on
      settings: AttributesFormatString=Sample time: %<SampleTime>
  PI_Daw_Out : Outport
  wires:
  Unary Minus/1 -> Saturation Dynamic/3
  Unit Delay/1 -> DiscreteAntiWindup/1(controlled_signal)
  P/1 -> Product1/3
  Discrete-Time Integrator/1 -> Add2/1
  ResetExt/1 -> Logical Operator/1, Discrete-Time Integrator/2
  Saturation Dynamic/1 -> PI_Daw_Out/1
  Product1/1 -> Add2/2
  Error/1 -> Product1/2, DiscreteAntiWindup/3(error)
  OutputLimit/1 -> Unary Minus/1, Saturation Dynamic/1, Abs/1
  Add2/1 -> Saturation Dynamic/2, Unit Delay/1  "FD_T_mot_ref_unsat"
  Abs/1 -> DiscreteAntiWindup/2("saturation_limit ")
  DiscreteAntiWindup/1(error_aw) -> Product2/1
  Product2/1 -> Discrete-Time Integrator/1
  I/1 -> Product2/2
  Logical Operator/1 -> Product1/1

== system FieldOrientedControl_Model/Inverter and Motor - Plant Model/Inverter/3phase converter ==
  g : Inport
  Converter (Three-Phase) : ee_lib/Semiconductors & Converters/Converters/Converter (Three-Phase)  port_option=ee.enum.threePhasePort.composite  fidelity_option=ee.enum.converters.fidelity.detailed  device_type=ee.enum.converters.switchingdevice.ideal  showThermalPort=false  K=0  Vth=0.5 V  Vgt=1 V  Vgt_off=-1 V  Ih=1 A  Vf=0.8 V  Ron=0.001 Ohm  Rds=0.001 Ohm  Goff=1e-6 1/Ohm  Eon_scalar=22.86e-3 J  Eoff_scalar=17.14e-3 J  Eoff_natural_commutation=10e-3 J  Voff=300 V  Iout_scalar=600 A  onCurrentMeasDelay=0 s  useCurrentFromPreviousCycle=false  useVoltageFromPreviousCycle=false  diode_param=ee.enum.converters.protectiondiode.none  diode_Vf=0.8 V  diode_Ron=0.001 Ohm  diode_Goff=1e-5 1/Ohm  diode_C=50 nF  diode_iRM=-235 A  diode_iF=300 A  diode_idot=-50 A/us  diode_trr_param=ee.enum.converters.diodetrr.trr_factor  diode_trr_factor=3  diode_trr=15 us  diode_Qrr=1500 s*uA  diode_rec_loss_model=ee.enum.diode.reverseRecoveryModel.fixed  diode_ErecVal=0 J  diode_scaleWithIandV=false  diode_ErecMat=zeros(2, 3) J  diode_TjrecVec=[298.15, 398.15] K  diode_IfrecVec=[.1, 1, 10] A  diode_IrecVal=10 A  diode_VrecVal=10 V  diode_tFilter=1 / 1000 / 100 s  thermal_network_parameterization=ee.enum.thermalNetworkTopology.external  Rth=[.08, .5] K/W  Rth_Cauer=[.08, .1, .5] K/W  Rth_Foster=[.08, .14, .22, .16] K/W  thermal_mass_parameterization=ee.enum.thermalNetwork.timeconstant  thermal_mass=[.01, .5] J/K  thermal_mass_Cauer=[.01, .1, .5] J/K  thermal_mass_Foster=[.001, .005, .05, .5] J/K  thermal_time_constant=[.001, .2] s  thermal_time_constant_Cauer=[.001, .1, .2] s  thermal_time_constant_Foster=[7e-05, .0007, .01, .08] s  thermal_mass_initial_temperatures=[25, 25] degC  thermal_mass_initial_temperatures_Cauer=[25, 25, 25] degC  junction_thermal_mass=0.01 J/K  Tvec_initial_Foster=[25, 25, 25, 25] degC  snubber_type=ee.enum.converters.snubber.exclude  Cs=1e-7 F  Rs=0.1 Ohm  Vce_loss=[0, 150, 300] V
  Demux : Demux  Outputs=6
  Scope : Scope  NumInputPorts=6
  Simulink-PS Converter{,1..5} (6 alike) : nesl_utility/Simulink-PS Converter  PhysicalDomain=network_engine_domain  SubClassName=ps_input  LeftPortType=input  RightPortType=output  PseudoPeriodic=off  Frequencies=[]  NoiseDistribution=none  NoiseParameters=[]  Unit=1  AffineConversion=off  FilteringAndDerivatives=provide  SimscapeFilterOrder=1  InputFilterTimeConstant=0.001  UdotUserProvided=0
  Six-Pulse Gate Multiplexer : ee_lib/Semiconductors & Converters/Converters/Six-Pulse Gate Multiplexer  port_option=ee.enum.controlport.ps
  + : PMIOPort  Side=Right
  ~ : PMIOPort  Port=2  Side=Left
  - : PMIOPort  Port=3  Side=Right
  wires:
  g/1 -> Demux/1
  Demux/1 -> Scope/1, Simulink-PS Converter/1
  Demux/2 -> Scope/2, Simulink-PS Converter1/1
  Demux/3 -> Scope/3, Simulink-PS Converter2/1
  Demux/4 -> Scope/4, Simulink-PS Converter3/1
  Demux/6 -> Scope/6, Simulink-PS Converter5/1
  Demux/5 -> Scope/5, Simulink-PS Converter4/1
  connections:
  Simulink-PS Converter/RConn1 -- Six-Pulse Gate Multiplexer/LConn1
  Converter (Three-Phase)/RConn2 -- -/RConn1
  Converter (Three-Phase)/RConn1 -- +/RConn1
  Converter (Three-Phase)/LConn2 -- ~/RConn1
  Six-Pulse Gate Multiplexer/RConn1 -- Converter (Three-Phase)/LConn1
  Simulink-PS Converter1/RConn1 -- Six-Pulse Gate Multiplexer/LConn2
  Simulink-PS Converter2/RConn1 -- Six-Pulse Gate Multiplexer/LConn3
  Simulink-PS Converter3/RConn1 -- Six-Pulse Gate Multiplexer/LConn4
  Simulink-PS Converter4/RConn1 -- Six-Pulse Gate Multiplexer/LConn5
  Simulink-PS Converter5/RConn1 -- Six-Pulse Gate Multiplexer/LConn6

== system FieldOrientedControl_Model/Inverter and Motor - Plant Model/Inverter/6-pulse PWM generator ==
  ModWave : Inport
  Data Type Conversion : DataTypeConversion  SaturateOnIntegerOverflow=off  RndMeth=Floor
  Mux : Mux  Inputs=2
  NOT : Logic  Operator=NOT  IconShape=distinctive  AllPortsSameDT=off  OutDataTypeStr=boolean
  Relay : Relay
  Repeating Sequence Interpolated : simulink/Sources/Repeating Sequence Interpolated  OutValues=[0 1 0 -1 0].'  TimeValues=0.25/fs*[0 1 2 3 4].'  LookUpMeth=Interpolation-Use End Values  tsamp=Ts  OutMin=[]  OutMax=[]  OutDataTypeStr=double  OutputDataTypeScalingMode=double  OutDataType=fixdt(0,8)  OutScaling=2^-10
  Scope : Scope
  Scope1 : Scope  NumInputPorts=4
  Selector : Selector  InputPortWidth=6  IndexOptions=Index vector (dialog)  Indices=[1 4 2 5 3 6]  OutputSizes=1
  Sum : Sum  Inputs=|+-
  g : Outport
  wires:
  Selector/1 -> g/1
  Mux/1 -> Selector/1
  Repeating Sequence Interpolated/1 -> Scope/1, Sum/2  "carrier"
  Sum/1 -> Scope1/2, Relay/1
  Relay/1 -> Scope1/3, Mux/1, NOT/1
  NOT/1 -> Scope1/4, Data Type Conversion/1
  ModWave/1 -> Scope1/1, Sum/1
  Data Type Conversion/1 -> Mux/2

== system FieldOrientedControl_Model/Inverter and Motor - Plant Model/Inverter/Scale ==
  duty_abc : Inport
  Constant : Constant  Value=0  OutDataTypeStr=double  SampleTime=Ts
  Data Type Conversion : DataTypeConversion  OutDataTypeStr=double  RndMeth=Simplest  SaturateOnIntegerOverflow=off
  Gain : Gain
  Rate Transition : RateTransition  OutPortSampleTime=Ts
  Sum : Sum  Inputs=|++
  ModWave : Outport
  wires:
  Sum/1 -> Gain/1
  Constant/1 -> Sum/2
  duty_abc/1 -> Data Type Conversion/1
  Gain/1 -> Rate Transition/1
  Rate Transition/1 -> ModWave/1  "ModWave"
  Data Type Conversion/1 -> Sum/1

== system FieldOrientedControl_Model/FOC_Ctrl/FOC_Control/Current Transformation/Clark Transformation ==
  i_a_meas_[A] : Inport
  i_b_meas_[A] : Inport  Port=2
  1/sqrt(3) : Constant  Value=1/sqrt(3)  OutDataTypeStr=single
  2/sqrt(3) : Constant  Value=2/sqrt(3)  OutDataTypeStr=single
  Add : Sum
  Product : Product
  Product1 : Product
  i_x_[A] : Outport
  i_y_[A] : Outport  Port=2
  wires:
  1/sqrt(3)/1 -> Product/2
  i_a_meas_[A]/1 -> Product/1, i_x_[A]/1
  i_b_meas_[A]/1 -> Product1/1
  2/sqrt(3)/1 -> Product1/2
  Product/1 -> Add/1
  Product1/1 -> Add/2
  Add/1 -> i_y_[A]/1

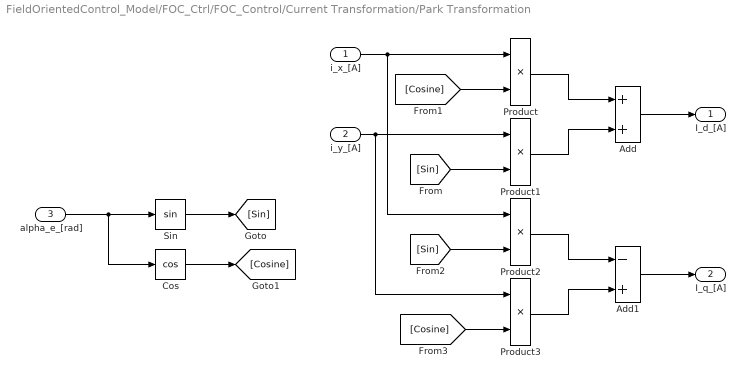
== system FieldOrientedControl_Model/FOC_Ctrl/FOC_Control/Current Transformation/Park Transformation ==
  i_x_[A] : Inport
  i_y_[A] : Inport  Port=2
  alpha_e_[rad] : Inport  Port=3
  Add : Sum
  Add1 : Sum  Inputs=-+  AccumDataTypeStr=double
  Cos : Trigonometry  Operator=cos
  Product : Product
  Product1 : Product
  Product2 : Product  OutDataTypeStr=double
  Product3 : Product  OutDataTypeStr=double
  Sin : Trigonometry
  I_d_[A] : Outport
  I_q_[A] : Outport  Port=2
  wires:
  alpha_e_[rad]/1 -> Cos/1, Sin/1
  Sin/1 -> [Sin]
  Cos/1 -> [Cosine]
  i_x_[A]/1 -> Product2/1, Product/1
  [Cosine] -> Product/2
  [Sin] -> Product1/2
  [Sin] -> Product2/2
  [Cosine] -> Product3/2
  i_y_[A]/1 -> Product3/1, Product1/1
  Product/1 -> Add/1
  Product1/1 -> Add/2
  Product2/1 -> Add1/1
  Product3/1 -> Add1/2
  Add/1 -> I_d_[A]/1
  Add1/1 -> I_q_[A]/1

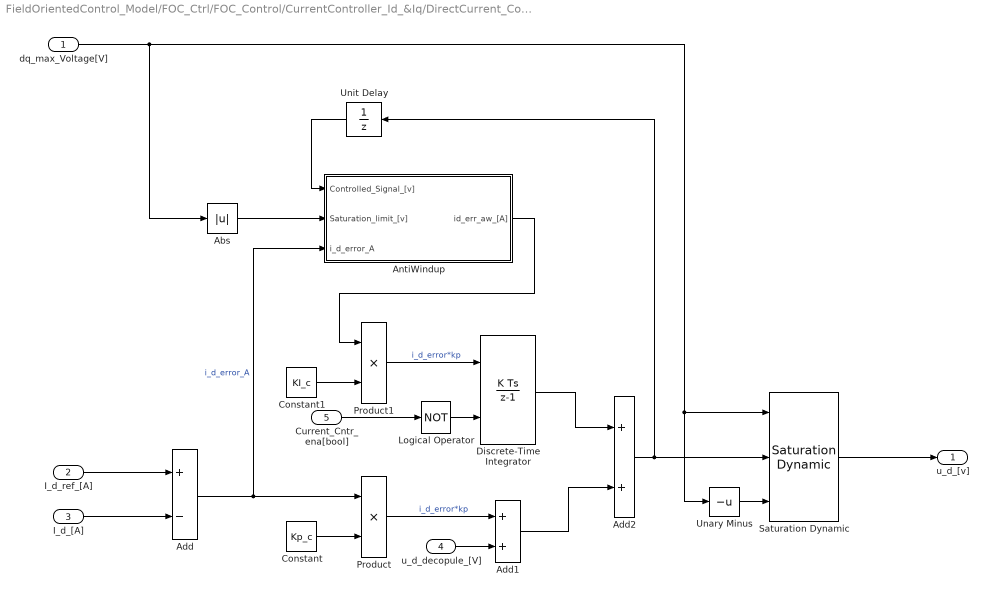
== system FieldOrientedControl_Model/FOC_Ctrl/FOC_Control/CurrentController_Id_&Iq/DirectCurrent_Control ==
  dq_max_Voltage[V] : Inport
  I_d_ref_[A] : Inport  Port=2
  I_d_[A] : Inport  Port=3
  u_d_decopule_[V] : Inport  Port=4
  Current_Cntr_ena[bool] : Inport  Port=5
  Abs : Abs  SaturateOnIntegerOverflow=off
  Add : Sum  Inputs=+-
  Add1 : Sum
  Add2 : Sum
  AntiWindup : Subsystem
  Constant : Constant  Value=Kp_c
  Constant1 : Constant  Value=KI_c
  Discrete-Time Integrator : DiscreteIntegrator  ExternalReset=level  SampleTime=-1  ICPrevOutput=DiscIntNeverNeededParam  ICPrevScaledInput=DiscIntNeverNeededParam
  Logical Operator : Logic  Operator=NOT  AllPortsSameDT=off  OutDataTypeStr=boolean
  Product : Product
  Product1 : Product
  Saturation Dynamic : simulink/Discontinuities/Saturation Dynamic  OutMin=[]  OutMax=[]  OutDataTypeStr=Inherit: Same as second input  OutDataType=fixdt(1, 16)  OutScaling=2^-10  DoSatur=off
  Unary Minus : UnaryMinus
  Unit Delay : UnitDelay  SampleTime=-1  HasFrameUpgradeWarning=on
  u_d_[v] : Outport
  wires:
  I_d_ref_[A]/1 -> Add/1
  I_d_[A]/1 -> Add/2
  Add/1 -> AntiWindup/3(i_d_error_A), Product/1  "i_d_error_A"
  Constant/1 -> Product/2
  Product/1 -> Add1/1  "i_d_error*kp"
  u_d_decopule_[V]/1 -> Add1/2
  Constant1/1 -> Product1/2
  Product1/1 -> Discrete-Time Integrator/1  "i_d_error*kp"
  Current_Cntr_ena[bool]/1 -> Logical Operator/1
  Logical Operator/1 -> Discrete-Time Integrator/2
  Discrete-Time Integrator/1 -> Add2/1
  Add1/1 -> Add2/2
  Add2/1 -> Saturation Dynamic/2, Unit Delay/1
  Unary Minus/1 -> Saturation Dynamic/3
  dq_max_Voltage[V]/1 -> Abs/1, Unary Minus/1, Saturation Dynamic/1
  Saturation Dynamic/1 -> u_d_[v]/1
  Unit Delay/1 -> AntiWindup/1(Controlled_Signal_[v])
  Abs/1 -> AntiWindup/2(Saturation_limit_[v])
  AntiWindup/1(id_err_aw_[A]) -> Product1/1

== system FieldOrientedControl_Model/FOC_Ctrl/FOC_Control/CurrentController_Id_&Iq/Maximum_dq_VoltageValue ==
  U_bat_[V] : Inport
  1/sqrt(3) : Constant  Value=dq_voltage_ratio
  Product : Product
  max_dq_Voltage[V] : Outport
  wires:
  U_bat_[V]/1 -> Product/1
  1/sqrt(3)/1 -> Product/2
  Product/1 -> max_dq_Voltage[V]/1  "max_dq_Voltage_V"

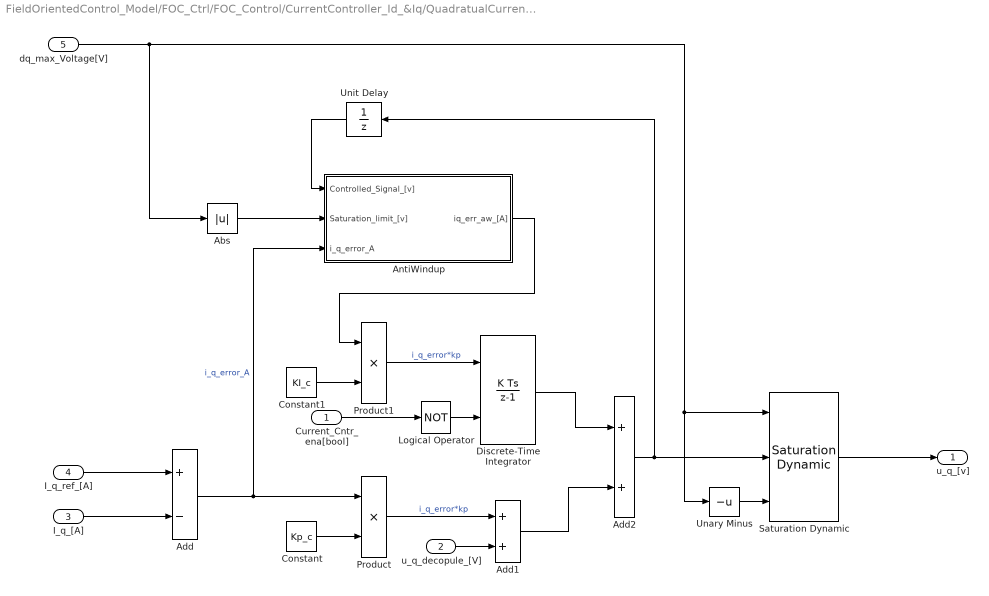
== system FieldOrientedControl_Model/FOC_Ctrl/FOC_Control/CurrentController_Id_&Iq/QuadratualCurrent_Control ==
  Current_Cntr_ena[bool] : Inport
  u_q_decopule_[V] : Inport  Port=2
  I_q_[A] : Inport  Port=3
  I_q_ref_[A] : Inport  Port=4
  dq_max_Voltage[V] : Inport  Port=5
  Abs : Abs  SaturateOnIntegerOverflow=off
  Add : Sum  Inputs=+-
  Add1 : Sum
  Add2 : Sum
  AntiWindup : Subsystem
  Constant : Constant  Value=Kp_c
  Constant1 : Constant  Value=KI_c
  Discrete-Time Integrator : DiscreteIntegrator  ExternalReset=level  SampleTime=-1  ICPrevOutput=DiscIntNeverNeededParam  ICPrevScaledInput=DiscIntNeverNeededParam
  Logical Operator : Logic  Operator=NOT  AllPortsSameDT=off  OutDataTypeStr=boolean
  Product : Product
  Product1 : Product
  Saturation Dynamic : simulink/Discontinuities/Saturation Dynamic  OutMin=[]  OutMax=[]  OutDataTypeStr=Inherit: Same as second input  OutDataType=fixdt(1, 16)  OutScaling=2^-10  DoSatur=off
  Unary Minus : UnaryMinus
  Unit Delay : UnitDelay  SampleTime=-1  HasFrameUpgradeWarning=on
  u_q_[v] : Outport
  wires:
  AntiWindup/1(iq_err_aw_[A]) -> Product1/1
  Abs/1 -> AntiWindup/2(Saturation_limit_[v])
  Unit Delay/1 -> AntiWindup/1(Controlled_Signal_[v])
  Saturation Dynamic/1 -> u_q_[v]/1
  dq_max_Voltage[V]/1 -> Saturation Dynamic/1, Unary Minus/1, Abs/1
  Unary Minus/1 -> Saturation Dynamic/3
  Add2/1 -> Unit Delay/1, Saturation Dynamic/2
  Add1/1 -> Add2/2
  Discrete-Time Integrator/1 -> Add2/1
  Logical Operator/1 -> Discrete-Time Integrator/2
  Current_Cntr_ena[bool]/1 -> Logical Operator/1
  Product1/1 -> Discrete-Time Integrator/1  "i_q_error*kp"
  Constant1/1 -> Product1/2
  u_q_decopule_[V]/1 -> Add1/2
  Product/1 -> Add1/1  "i_q_error*kp"
  Constant/1 -> Product/2
  Add/1 -> Product/1, AntiWindup/3(i_q_error_A)  "i_q_error_A"
  I_q_[A]/1 -> Add/2
  I_q_ref_[A]/1 -> Add/1

== system FieldOrientedControl_Model/FOC_Ctrl/FOC_Control/CurrentController_Id_&Iq/Voltage Decopling ==
  I_d_[A] : Inport
  w_e_[rad/s] : Inport  Port=2
  I_q_[A] : Inport  Port=3
  Enable : EnablePort
  Add : Sum  AccumDataTypeStr=single
  Constant : Constant  Value=L_q  VectorParams1D=off
  Constant1 : Constant  Value=L_q
  Constant2 : Constant  Value=Psi_p
  Constant3 : Constant  Value=-1
  Product : Product  Inputs=4  OutDataTypeStr=single
  Product1 : Product  OutDataTypeStr=single
  Product2 : Product  OutDataTypeStr=single
  u_d_decopule_[V] : Outport
  u_q_decopule_[V] : Outport  Port=2
  wires:
  I_q_[A]/1 -> Product/1
  w_e_[rad/s]/1 -> Product2/1, Product/2
  Constant/1 -> Product/3
  Constant3/1 -> Product/4
  I_d_[A]/1 -> Product1/1
  Constant1/1 -> Product1/2
  Product1/1 -> Add/1
  Constant2/1 -> Add/2
  Add/1 -> Product2/2
  Product/1 -> u_d_decopule_[V]/1  "u_d_decopled_V"
  Product2/1 -> u_q_decopule_[V]/1  "u_d_decopled_V"

== system FieldOrientedControl_Model/FOC_Ctrl/FOC_Control/SVPWM/SafeDevision ==
  U_bat_[v] : Inport
  Compare To Constant : simulink/Logic and Bit Operations/Compare To Constant  relop===  const=0  OutDataTypeStr=boolean
  Constant : Constant  Value=1e-6
  Switch : Switch  Criteria=u2 ~= 0  SaturateOnIntegerOverflow=off  InputSameDT=off
  U_bat_safe_div_[v] : Outport
  wires:
  Switch/1 -> U_bat_safe_div_[v]/1
  Compare To Constant/1 -> Switch/2
  U_bat_[v]/1 -> Compare To Constant/1, Switch/3
  Constant/1 -> Switch/1

== system FieldOrientedControl_Model/FOC_Ctrl/FOC_Control/Voltage Transfromation/Inverse Clark Transformation  ==
  u_x_[v] : Inport
  u_y_[v] : Inport  Port=2
  1/2 : Constant  Value=1/2
  Add : Sum  Inputs=-+
  Add1 : Sum  Inputs=--
  Product : Product
  Product1 : Product
  sqrt(3)/2 : Constant  Value=sqrt(3)/2
  u_ref_a_[v] : Outport
  u_ref_b_[v] : Outport  Port=2
  u_ref_c_[v] : Outport  Port=3
  wires:
  u_x_[v]/1 -> Product/1, u_ref_a_[v]/1
  1/2/1 -> Product/2
  Product/1 -> Add1/1, Add/1
  u_y_[v]/1 -> Product1/1
  sqrt(3)/2/1 -> Product1/2
  Add/1 -> u_ref_b_[v]/1
  Product1/1 -> Add1/2, Add/2
  Add1/1 -> u_ref_c_[v]/1

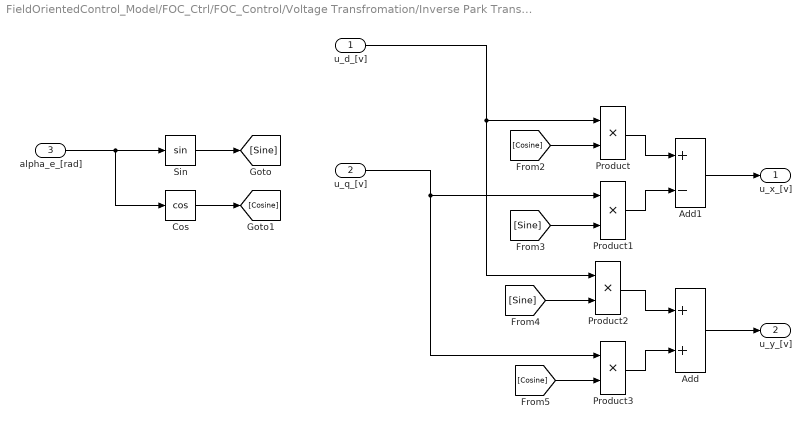
== system FieldOrientedControl_Model/FOC_Ctrl/FOC_Control/Voltage Transfromation/Inverse Park Transformation ==
  u_d_[v] : Inport
  u_q_[v] : Inport  Port=2
  alpha_e_[rad] : Inport  Port=3
  Add : Sum
  Add1 : Sum  Inputs=+-
  Cos : Trigonometry  Operator=cos
  Product{,1..3} (4 alike) : Product
  Sin : Trigonometry
  u_x_[v] : Outport
  u_y_[v] : Outport  Port=2
  wires:
  alpha_e_[rad]/1 -> Cos/1, Sin/1
  Sin/1 -> [Sine]
  Cos/1 -> [Cosine]
  u_d_[v]/1 -> Product2/1, Product/1
  [Cosine] -> Product/2
  u_q_[v]/1 -> Product3/1, Product1/1
  [Sine] -> Product1/2
  [Sine] -> Product2/2
  [Cosine] -> Product3/2
  Product2/1 -> Add/1
  Product3/1 -> Add/2
  Product1/1 -> Add1/2
  Product/1 -> Add1/1
  Add/1 -> u_y_[v]/1
  Add1/1 -> u_x_[v]/1

== system FieldOrientedControl_Model/FOC_Ctrl/FrequencyControl_PI/PI regulator/DiscreteAntiWindup ==
  note: Saturation Detection
  note: Anti-Windup in Saturation
  controlled_signal : Inport
  "saturation_limit " : Inport  Port=2
  error : Inport  Port=3
  Abs : Abs  RndMeth=Simplest
  Abs1 : Abs  RndMeth=Simplest
  Constant : Constant  Value=0  OutDataTypeStr=single
  OR : Logic  Operator=OR  AllPortsSameDT=off  OutDataTypeStr=boolean
  Product : Product  RndMeth=Simplest  SaturateOnIntegerOverflow=on
  Product1 : Product  RndMeth=Simplest  SaturateOnIntegerOverflow=on
  Relational Operator : RelationalOperator  Operator=<  OutDataTypeStr=boolean  RndMeth=Simplest  InputSameDT=off
  Relational Operator1 : RelationalOperator  Operator=<  OutDataTypeStr=boolean  RndMeth=Simplest  InputSameDT=off
  error_aw : Outport
  wires:
  Relational Operator1/1 -> OR/2
  Constant/1 -> Relational Operator1/2
  Product1/1 -> Relational Operator1/1
  Product/1 -> error_aw/1
  error/1 -> Product/2, Product1/2
  OR/1 -> Product/1
  Relational Operator/1 -> OR/1
  Abs/1 -> Relational Operator/1
  Abs1/1 -> Relational Operator/2
  "saturation_limit "/1 -> Abs1/1
  controlled_signal/1 -> Abs/1, Product1/1

== system FieldOrientedControl_Model/FOC_Ctrl/FOC_Control/CurrentController_Id_&Iq/DirectCurrent_Control/AntiWindup ==
  Controlled_Signal_[v] : Inport
  Saturation_limit_[v] : Inport  Port=2
  i_d_error_A : Inport  Port=3
  Abs : Abs  SaturateOnIntegerOverflow=off
  Product : Product
  Relational Operator : RelationalOperator  Operator=<  OutDataTypeStr=boolean  RndMeth=Simplest  InputSameDT=off
  id_err_aw_[A] : Outport
  wires:
  Controlled_Signal_[v]/1 -> Abs/1
  Abs/1 -> Relational Operator/1
  Saturation_limit_[v]/1 -> Relational Operator/2
  Relational Operator/1 -> Product/1
  i_d_error_A/1 -> Product/2
  Product/1 -> id_err_aw_[A]/1

== system FieldOrientedControl_Model/FOC_Ctrl/FOC_Control/CurrentController_Id_&Iq/QuadratualCurrent_Control/AntiWindup ==
  Controlled_Signal_[v] : Inport
  Saturation_limit_[v] : Inport  Port=2
  i_q_error_A : Inport  Port=3
  Abs : Abs  SaturateOnIntegerOverflow=off
  Product : Product
  Relational Operator : RelationalOperator  Operator=<  OutDataTypeStr=boolean  RndMeth=Simplest  InputSameDT=off
  iq_err_aw_[A] : Outport
  wires:
  Product/1 -> iq_err_aw_[A]/1
  i_q_error_A/1 -> Product/2
  Relational Operator/1 -> Product/1
  Saturation_limit_[v]/1 -> Relational Operator/2
  Abs/1 -> Relational Operator/1
  Controlled_Signal_[v]/1 -> Abs/1

== stateflow chart FieldOrientedControl_Model/FOC_Ctrl/FOC_Control/SVPWM/Chart ==
  note: ?
  (default) -> (junction 10)
  (junction 10) -> (junction 12) [order 1] : [sector == 1 | sector == 4]{
      | duty_a=duty_offset + duty_offset*(u_a - u_c);
      | duty_b=duty_offset + duty_offset*(2*u_b - u_a - u_c);
      | duty_c=duty_offset + duty_offset*(u_c - u_a);
      | }
  (junction 10) -> (junction 14) [order 2]
  (junction 14) -> (junction 15) [order 1] : [sector == 2 | sector == 5]{
      | duty_a=duty_offset + duty_offset*(2*u_a - u_b - u_c);
      | duty_b=duty_offset + duty_offset*(u_b - u_c);
      | duty_c=duty_offset + duty_offset*(u_c - u_b);
      | }
  (junction 14) -> (junction 18) [order 2]
  (junction 18) -> (junction 20) : [sector == 3 | sector == 6]{
      | duty_a=duty_offset + duty_offset*(u_a - u_b);
      | duty_b=duty_offset + duty_offset*(u_b - u_a);
      | duty_c=duty_offset + duty_offset*(2*u_c - u_a - u_b);
      | }
  data: duty_offset input; u_a input; u_b input; u_c input; sector input; duty_a output; duty_b output; duty_c output

== stateflow chart FieldOrientedControl_Model/FOC_Ctrl/FOC_Control/SVPWM/voltage_sector_detection ==
  (default) -> (junction 4)
  (junction 4) -> (junction 19) [order 2]
  (junction 4) -> (junction 6) [order 1] : [u_a>=u_b]
  (junction 19) -> (junction 22)
  (junction 6) -> (junction 7) [order 1] : [u_c>=u_a]{sector = 5 }
  (junction 22) -> (junction 24) [order 1] : [u_a>=u_c]{sector = 2 }
  (junction 6) -> (junction 11) [order 2]
  (junction 22) -> (junction 26) [order 2]
  (junction 11) -> (junction 12) [order 1] : [u_c>=u_b]{sector = 6 }
  (junction 26) -> (junction 28) [order 1] : [u_b>=u_c]{sector = 3 }
  (junction 11) -> (junction 15) [order 2]
  (junction 26) -> (junction 30) [order 2]
  (junction 15) -> (junction 17) : {sector = 1 }
  (junction 30) -> (junction 32) : {sector = 4}
  data: u_a input; u_b input; u_c input; sector output
